simulink model "Day13"  (R2024b)
settings: Solver=VariableStepAuto  StartTime=0.0  StopTime=10.0  RelTol=1e-3
settings Model: Creator=jun_mac  LastModifiedBy=jun_mac

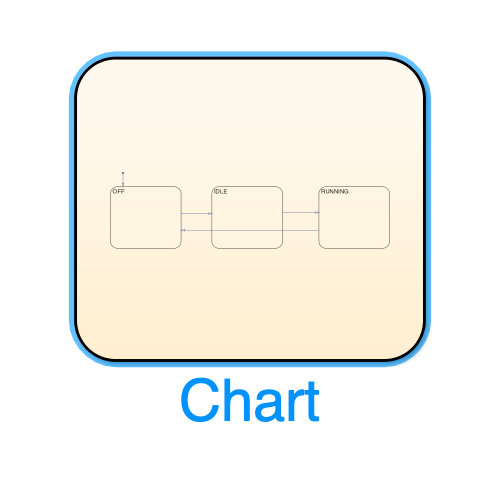
[thumbnail: Simulink's stored preview of the top-level diagram]
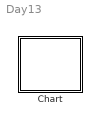
== system Day13 ==
  Chart : Stateflow chart  TreatAsAtomicUnit=on

== stateflow chart Day13/Chart ==
  state OFF
  state IDLE
  state RUNNING
  (default) -> OFF
  IDLE -> RUNNING
  OFF -> IDLE
  RUNNING -> OFF
